simulink model "RealHardwareControlSample"  (R2015a)
settings: configuration reference "SIMULATION_CONFIGURATION" (kept outside this file)
settings Model: Creator=moritz  LastModifiedBy=moritz
settings ConfigSetRef: SourceLocation=Base Workspace

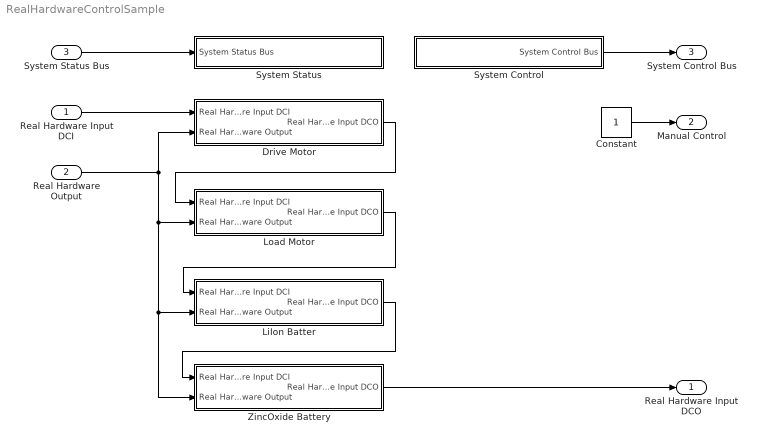
== system RealHardwareControlSample ==
  Real Hardware Input DCI : Inport  OutDataTypeStr=Bus: HARDWARE_IO_INPUT_BUS  BusOutputAsStruct=on
  Real Hardware Output : Inport  Port=2  OutDataTypeStr=Bus: HARDWARE_IO_OUTPUT_BUS  BusOutputAsStruct=on
  System Status Bus : Inport  Port=3  OutDataTypeStr=Bus: SYSTEM_STATUS_BUS  BusOutputAsStruct=on
  Constant : Constant  OutDataTypeStr=boolean
  Drive Motor : Subsystem
  LiIon Batter : Subsystem
  Load Motor : Subsystem
  System Control : Subsystem
  System Status : Subsystem
  ZincOxide Battery : Subsystem
  Real Hardware Input DCO : Outport  OutDataTypeStr=Bus: HARDWARE_IO_INPUT_BUS  BusOutputAsStruct=on
  Manual Control : Outport  Port=2
  System Control Bus : Outport  Port=3  OutDataTypeStr=Bus: SYSTEM_CONTROL_BUS  BusOutputAsStruct=on
  wires:
  Constant/1 -> Manual Control/1
  Real Hardware Input DCI/1 -> Drive Motor/1(Real Hardware Input DCI)
  Real Hardware Output/1 -> ZincOxide Battery/2(Real Hardware Output), LiIon Batter/2(Real Hardware Output), Load Motor/2(Real Hardware Output), Drive Motor/2(Real Hardware Output)
  System Status Bus/1 -> System Status/1(System Status Bus)
  Drive Motor/1(Real Hardware Input DCO) -> Load Motor/1(Real Hardware Input DCI)
  Load Motor/1(Real Hardware Input DCO) -> LiIon Batter/1(Real Hardware Input DCI)
  LiIon Batter/1(Real Hardware Input DCO) -> ZincOxide Battery/1(Real Hardware Input DCI)
  ZincOxide Battery/1(Real Hardware Input DCO) -> Real Hardware Input DCO/1
  System Control/1(System Control Bus) -> System Control Bus/1

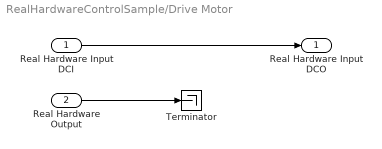
== system RealHardwareControlSample/Drive Motor ==
  Real Hardware Input DCI : Inport
  Real Hardware Output : Inport  Port=2
  Terminator : Terminator
  Real Hardware Input DCO : Outport
  wires:
  Real Hardware Input DCI/1 -> Real Hardware Input DCO/1
  Real Hardware Output/1 -> Terminator/1

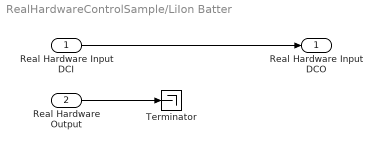
== system RealHardwareControlSample/LiIon Batter ==
  Real Hardware Input DCI : Inport
  Real Hardware Output : Inport  Port=2
  Terminator : Terminator
  Real Hardware Input DCO : Outport
  wires:
  Real Hardware Input DCI/1 -> Real Hardware Input DCO/1
  Real Hardware Output/1 -> Terminator/1

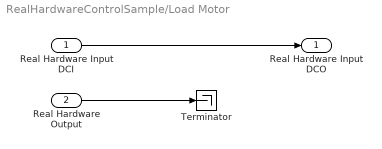
== system RealHardwareControlSample/Load Motor ==
  Real Hardware Input DCI : Inport
  Real Hardware Output : Inport  Port=2
  Terminator : Terminator
  Real Hardware Input DCO : Outport
  wires:
  Real Hardware Input DCI/1 -> Real Hardware Input DCO/1
  Real Hardware Output/1 -> Terminator/1

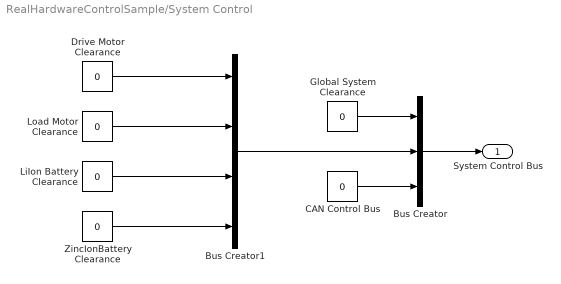
== system RealHardwareControlSample/System Control ==
  Bus Creator : BusCreator  Inputs=3
  Bus Creator1 : BusCreator
  CAN Control Bus : Constant  Value=0  OutDataTypeStr=Bus: CAN_CONTROL_BUS
  Drive Motor Clearance : Constant  Value=0  OutDataTypeStr=boolean
  Global System Clearance : Constant  Value=0  OutDataTypeStr=boolean
  LiIon Battery Clearance : Constant  Value=0  OutDataTypeStr=boolean
  Load Motor Clearance : Constant  Value=0  OutDataTypeStr=boolean
  ZincIonBattery Clearance : Constant  Value=0  OutDataTypeStr=boolean
  System Control Bus : Outport
  wires:
  Bus Creator/1 -> System Control Bus/1
  Global System Clearance/1 -> Bus Creator/1
  Bus Creator1/1 -> Bus Creator/2
  CAN Control Bus/1 -> Bus Creator/3
  Drive Motor Clearance/1 -> Bus Creator1/1
  Load Motor Clearance/1 -> Bus Creator1/2
  LiIon Battery Clearance/1 -> Bus Creator1/3
  ZincIonBattery Clearance/1 -> Bus Creator1/4

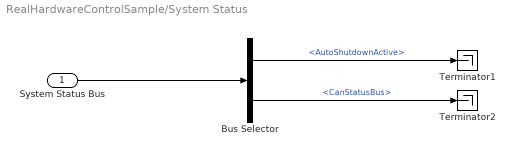
== system RealHardwareControlSample/System Status ==
  System Status Bus : Inport
  Bus Selector : BusSelector  OutputSignals=AutoShutdownActive,CanStatusBus
  Terminator1 : Terminator
  Terminator2 : Terminator
  wires:
  System Status Bus/1 -> Bus Selector/1
  Bus Selector/1 -> Terminator1/1  "<AutoShutdownActive>"
  Bus Selector/2 -> Terminator2/1  "<CanStatusBus>"

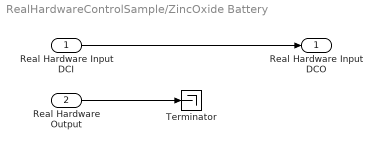
== system RealHardwareControlSample/ZincOxide Battery ==
  Real Hardware Input DCI : Inport
  Real Hardware Output : Inport  Port=2
  Terminator : Terminator
  Real Hardware Input DCO : Outport
  wires:
  Real Hardware Input DCI/1 -> Real Hardware Input DCO/1
  Real Hardware Output/1 -> Terminator/1
